simulink model "frFanA_20160929aSIM"  (R2013a)
settings: Solver=ode45  StartTime=0.0  StopTime=3  RelTol=1e-3
libraries: blockBEACON x7
settings Model: Creator=210023782  LastModifiedBy=210023782

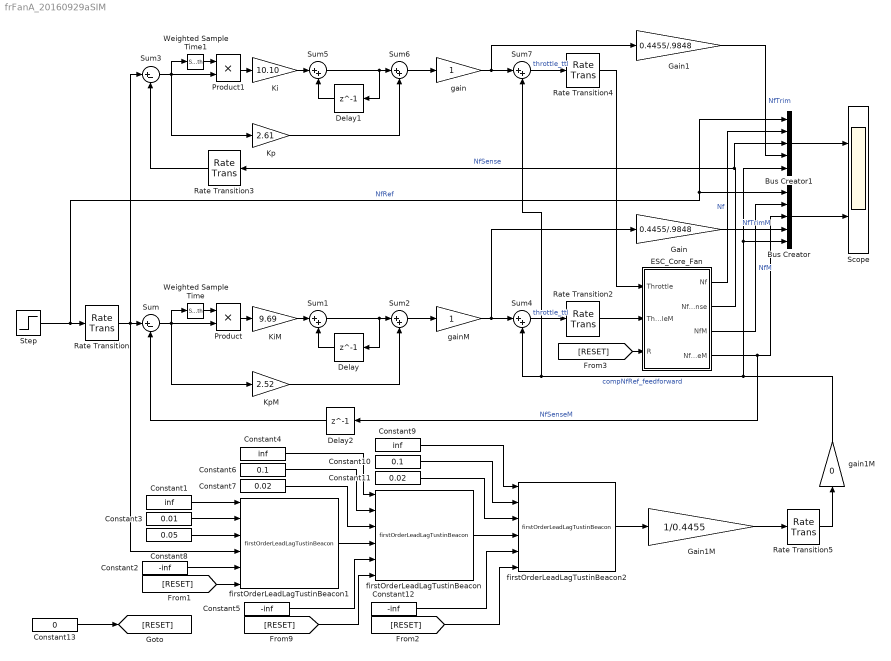
== system frFanA_20160929aSIM ==
  Bus Creator : BusCreator  Inputs=5
  Bus Creator1 : BusCreator  Inputs=5
  Constant1 : Constant  Value=inf
  Constant10 : Constant  Value=0.1
  Constant11 : Constant  Value=0.02
  Constant12 : Constant  Value=-inf
  Constant13 : Constant  Value=0
  Constant2 : Constant  Value=-inf
  Constant3 : Constant  Value=0.01
  Constant4 : Constant  Value=inf
  Constant5 : Constant  Value=-inf
  Constant6 : Constant  Value=0.1
  Constant7 : Constant  Value=0.02
  Constant8 : Constant  Value=0.05
  Constant9 : Constant  Value=inf
  Delay : Delay  DelayLength=1  InitialCondition=0
  Delay1 : Delay  DelayLength=1  InitialCondition=0
  Delay2 : Delay  DelayLength=1  InitialCondition=0  SampleTime=0.015
  ESC_Core_Fan : Subsystem
  Gain : Gain  Gain=0.4455/.9848
  Gain1 : Gain  Gain=0.4455/.9848
  Gain1M : Gain  Gain=1/0.4455
  Ki : Gain  Gain=10.10
  KiM : Gain  Gain=9.69
  Kp : Gain  Gain=2.61
  KpM : Gain  Gain=2.52
  Product : Product
  Product1 : Product
  Rate Transition{,2..5} (5 alike) : RateTransition  OutPortSampleTime=0.015
  Scope : Scope  NumInputPorts=2
      settings: ShowLegends=on  YMin=0.9975~-5  YMax=1.0175~5
  Step : Step  Time=0.1  SampleTime=0
  Sum : Sum  Inputs=|+-
  Sum{1..2,4..7} (6 alike) : Sum  Inputs=|++
  Sum3 : Sum  Inputs=|+-
  Weighted Sample Time : SampleTimeMath  TsampMathOp=Ts Only
  Weighted Sample Time1 : SampleTimeMath  TsampMathOp=Ts Only
  firstOrderLeadLagTustinBeacon : blockBEACON/firstOrderLeadLagTustinBeacon  T=.015
  firstOrderLeadLagTustinBeacon1 : blockBEACON/firstOrderLeadLagTustinBeacon  T=.015
  firstOrderLeadLagTustinBeacon2 : blockBEACON/firstOrderLeadLagTustinBeacon  T=.015
  gain : Gain
  gain1M : Gain  Gain=0
  gainM : Gain
  wires:
  Sum2/1 -> gainM/1
  Step/1 -> Bus Creator/1, Bus Creator1/1, Rate Transition/1  "NfRef"
  Delay2/1 -> Sum/2
  Delay/1 -> Sum1/2
  Sum1/1 -> Delay/1, Sum2/1
  Sum/1 -> KpM/1, Product/2, Weighted Sample Time/1
  Weighted Sample Time/1 -> Product/1
  Product/1 -> KiM/1
  KpM/1 -> Sum2/2
  Rate Transition2/1 -> ESC_Core_Fan/2(ThrottleM)
  KiM/1 -> Sum1/1
  Gain/1 -> Bus Creator/4  "NfTrimM"
  Constant6/1 -> firstOrderLeadLagTustinBeacon/2
  [RESET] -> firstOrderLeadLagTustinBeacon/6
  Constant5/1 -> firstOrderLeadLagTustinBeacon/5
  Constant4/1 -> firstOrderLeadLagTustinBeacon/1
  firstOrderLeadLagTustinBeacon1/1 -> firstOrderLeadLagTustinBeacon/4
  Constant7/1 -> firstOrderLeadLagTustinBeacon/3
  Constant3/1 -> firstOrderLeadLagTustinBeacon1/2
  [RESET] -> firstOrderLeadLagTustinBeacon1/6
  Constant2/1 -> firstOrderLeadLagTustinBeacon1/5
  Constant1/1 -> firstOrderLeadLagTustinBeacon1/1
  Rate Transition/1 -> Sum3/1, firstOrderLeadLagTustinBeacon1/4, Sum/1
  Constant8/1 -> firstOrderLeadLagTustinBeacon1/3
  firstOrderLeadLagTustinBeacon/1 -> firstOrderLeadLagTustinBeacon2/4
  Constant11/1 -> firstOrderLeadLagTustinBeacon2/3
  Constant9/1 -> firstOrderLeadLagTustinBeacon2/1
  Constant10/1 -> firstOrderLeadLagTustinBeacon2/2
  [RESET] -> firstOrderLeadLagTustinBeacon2/6
  Constant12/1 -> firstOrderLeadLagTustinBeacon2/5
  firstOrderLeadLagTustinBeacon2/1 -> Gain1M/1
  ESC_Core_Fan/3(NfM) -> Bus Creator/2  "NfM"
  ESC_Core_Fan/4(NfSenseM) -> Bus Creator/3, Delay2/1  "NfSenseM"
  gainM/1 -> Gain/1, Sum4/1
  Sum4/1 -> Rate Transition2/1  "throttle_ttl"
  Gain1M/1 -> Rate Transition5/1
  gain1M/1 -> Bus Creator1/5, Bus Creator/5, Sum4/2, Sum7/2  "compNfRef_feedforward"
  Sum6/1 -> gain/1
  Rate Transition3/1 -> Sum3/2
  Delay1/1 -> Sum5/2
  Sum5/1 -> Sum6/1, Delay1/1
  Sum3/1 -> Weighted Sample Time1/1, Product1/2, Kp/1
  Weighted Sample Time1/1 -> Product1/1
  Product1/1 -> Ki/1
  Kp/1 -> Sum6/2
  Ki/1 -> Sum5/1
  ESC_Core_Fan/2(NfSense) -> Bus Creator1/3, Rate Transition3/1  "NfSense"
  gain/1 -> Sum7/1, Gain1/1
  Sum7/1 -> Rate Transition4/1  "throttle_ttl"
  Rate Transition4/1 -> ESC_Core_Fan/1(Throttle)
  Bus Creator1/1 -> Scope/1
  Bus Creator/1 -> Scope/2
  ESC_Core_Fan/1(Nf) -> Bus Creator1/2  "Nf"
  Gain1/1 -> Bus Creator1/4  "NfTrim"
  Rate Transition5/1 -> gain1M/1
  Constant13/1 -> [RESET]
  [RESET] -> ESC_Core_Fan/3(R)

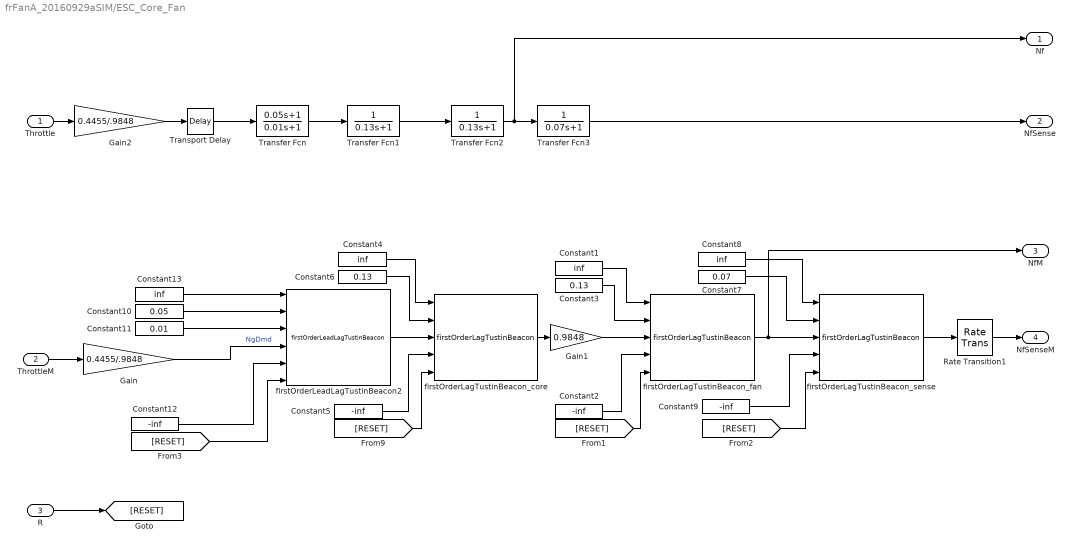
== system frFanA_20160929aSIM/ESC_Core_Fan ==
  Throttle : Inport
  ThrottleM : Inport  Port=2
  R : Inport  Port=3
  Constant{1,4,8,13} (4 alike) : Constant  Value=inf
  Constant10 : Constant  Value=0.05
  Constant11 : Constant  Value=0.01
  Constant{2,5,9,12} (4 alike) : Constant  Value=-inf
  Constant3 : Constant  Value=0.13
  Constant6 : Constant  Value=0.13
  Constant7 : Constant  Value=0.07
  Gain : Gain  Gain=0.4455/.9848
  Gain1 : Gain  Gain=0.9848
  Gain2 : Gain  Gain=0.4455/.9848
  Rate Transition1 : RateTransition
  Transfer Fcn : TransferFcn  Numerator=[0.05 1]  Denominator=[0.01 1]
  Transfer Fcn1 : TransferFcn  Denominator=[0.13 1]
  Transfer Fcn2 : TransferFcn  Denominator=[0.13 1]
  Transfer Fcn3 : TransferFcn  Denominator=[0.07 1]
  Transport Delay : TransportDelay  DelayTime=0.01
  firstOrderLagTustinBeacon_core : blockBEACON/firstOrderLagTustinBeacon  T=0.015
  firstOrderLagTustinBeacon_fan : blockBEACON/firstOrderLagTustinBeacon  T=0.015
  firstOrderLagTustinBeacon_sense : blockBEACON/firstOrderLagTustinBeacon  T=0.015
  firstOrderLeadLagTustinBeacon2 : blockBEACON/firstOrderLeadLagTustinBeacon  T=0.015
  Nf : Outport
  NfSense : Outport  Port=2
  NfM : Outport  Port=3
  NfSenseM : Outport  Port=4
  wires:
  ThrottleM/1 -> Gain/1
  Constant6/1 -> firstOrderLagTustinBeacon_core/2
  [RESET] -> firstOrderLagTustinBeacon_core/5
  Constant5/1 -> firstOrderLagTustinBeacon_core/4
  Constant4/1 -> firstOrderLagTustinBeacon_core/1
  Constant1/1 -> firstOrderLagTustinBeacon_fan/1
  Constant2/1 -> firstOrderLagTustinBeacon_fan/4
  [RESET] -> firstOrderLagTustinBeacon_fan/5
  Constant3/1 -> firstOrderLagTustinBeacon_fan/2
  firstOrderLagTustinBeacon_core/1 -> Gain1/1
  firstOrderLeadLagTustinBeacon2/1 -> firstOrderLagTustinBeacon_core/3
  Gain1/1 -> firstOrderLagTustinBeacon_fan/3
  firstOrderLagTustinBeacon_fan/1 -> NfM/1, firstOrderLagTustinBeacon_sense/3
  Constant7/1 -> firstOrderLagTustinBeacon_sense/2
  Constant8/1 -> firstOrderLagTustinBeacon_sense/1
  Constant9/1 -> firstOrderLagTustinBeacon_sense/4
  [RESET] -> firstOrderLagTustinBeacon_sense/5
  firstOrderLagTustinBeacon_sense/1 -> Rate Transition1/1
  Rate Transition1/1 -> NfSenseM/1
  Constant11/1 -> firstOrderLeadLagTustinBeacon2/3
  Constant13/1 -> firstOrderLeadLagTustinBeacon2/1
  Constant10/1 -> firstOrderLeadLagTustinBeacon2/2
  [RESET] -> firstOrderLeadLagTustinBeacon2/6
  Constant12/1 -> firstOrderLeadLagTustinBeacon2/5
  Gain/1 -> firstOrderLeadLagTustinBeacon2/4  "NgDmd"
  Throttle/1 -> Gain2/1
  Gain2/1 -> Transport Delay/1
  Transport Delay/1 -> Transfer Fcn/1
  Transfer Fcn/1 -> Transfer Fcn1/1
  Transfer Fcn1/1 -> Transfer Fcn2/1
  Transfer Fcn2/1 -> Nf/1, Transfer Fcn3/1
  Transfer Fcn3/1 -> NfSense/1
  R/1 -> [RESET]
